simulink model "Nonlinear_Adaptive_Backstepping_controller"  (R2021a)
settings: Solver=VariableStepAuto  StartTime=0.0  StopTime=50  RelTol=1e-3
libraries: simulink x2
settings Model: Creator=dell  LastModifiedBy=dell

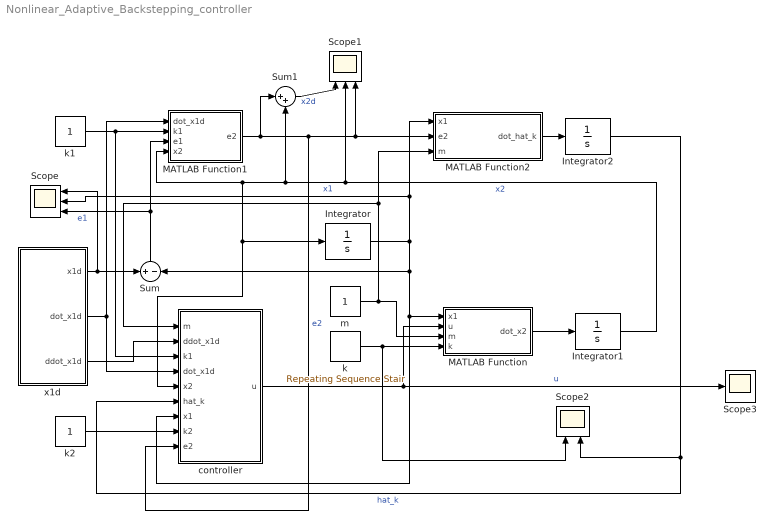
== system Nonlinear_Adaptive_Backstepping_controller ==
  Integrator : Integrator
  Integrator1 : Integrator
  Integrator2 : Integrator
  MATLAB Function : MATLAB Function  TreatAsAtomicUnit=on
  MATLAB Function1 : MATLAB Function  TreatAsAtomicUnit=on
  MATLAB Function2 : MATLAB Function  TreatAsAtomicUnit=on
  Scope : Scope  NumInputPorts=3
  Scope1 : Scope  NumInputPorts=3
  Scope2 : Scope  NumInputPorts=2
  Scope3 : Scope
  Sum : Sum  Inputs=+-
  Sum1 : Sum  Inputs=|++
  controller : MATLAB Function  TreatAsAtomicUnit=on
  k : simulink/Sources/Repeating Sequence Stair  OutValues=[3 1 4 1 5 9 2 6].'  tsamp=25  OutMin=[]  OutMax=[]  OutDataTypeStr=double  OutputDataTypeScalingMode=double  OutDataType=fixdt(0,8)  ConRadixGroup=Best Precision: Vector-wise  OutScaling=2^-12
  k1 : Constant
  k2 : Constant
  m : Constant
  x1d : Subsystem
  wires:
  Integrator/1 -> controller/7(x1), MATLAB Function/1(x1), Sum/2, Scope/2, MATLAB Function2/1(x1)  "x1"
  Integrator1/1 -> Scope1/2, Sum1/2, MATLAB Function1/4(x2), controller/5(x2), Integrator/1  "x2"
  m/1 -> MATLAB Function2/3(m), controller/1(m), MATLAB Function/3(m)
  k/1 -> Scope2/1, MATLAB Function/4(k)
  controller/1(u) -> Scope3/1, MATLAB Function/2(u)  "u"
  MATLAB Function/1(dot_x2) -> Integrator1/1
  x1d/1(x1d) -> Scope/1, Sum/1
  Sum/1 -> Scope/3, MATLAB Function1/3(e1)  "e1"
  x1d/2(dot_x1d) -> controller/4(dot_x1d), MATLAB Function1/1(dot_x1d)
  k1/1 -> MATLAB Function1/2(k1), controller/3(k1)
  MATLAB Function2/1(dot_hat_k) -> Integrator2/1
  Integrator2/1 -> Scope2/2, controller/6(hat_k)  "hat_k"
  MATLAB Function1/1(e2) -> Sum1/1, controller/9(e2), Scope1/3, MATLAB Function2/2(e2)  "e2"
  x1d/3(ddot_x1d) -> controller/2(ddot_x1d)
  k2/1 -> controller/8(k2)
  Sum1/1 -> Scope1/1  "x2d"

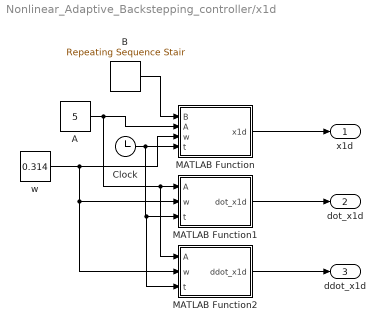
== system Nonlinear_Adaptive_Backstepping_controller/x1d ==
  A : Constant  Value=5
  B : simulink/Sources/Repeating Sequence Stair  OutValues=[0].'  tsamp=10  OutMin=[]  OutMax=[]  OutDataTypeStr=double  OutputDataTypeScalingMode=double  OutDataType=fixdt(0,8)  ConRadixGroup=Best Precision: Vector-wise  OutScaling=2^-12
  Clock : Clock
  MATLAB Function : MATLAB Function  TreatAsAtomicUnit=on
  MATLAB Function1 : MATLAB Function  TreatAsAtomicUnit=on
  MATLAB Function2 : MATLAB Function  TreatAsAtomicUnit=on
  w : Constant  Value=0.314
  x1d : Outport
  dot_x1d : Outport  Port=2
  ddot_x1d : Outport  Port=3
  wires:
  MATLAB Function/1(x1d) -> x1d/1
  Clock/1 -> MATLAB Function2/3(t), MATLAB Function1/3(t), MATLAB Function/4(t)
  B/1 -> MATLAB Function/1(B)
  A/1 -> MATLAB Function2/1(A), MATLAB Function1/1(A), MATLAB Function/2(A)
  w/1 -> MATLAB Function2/2(w), MATLAB Function1/2(w), MATLAB Function/3(w)
  MATLAB Function1/1(dot_x1d) -> dot_x1d/1
  MATLAB Function2/1(ddot_x1d) -> ddot_x1d/1

== matlab function Nonlinear_Adaptive_Backstepping_controller/controller ==
  data: m input; u output; ddot_x1d input; k1 input; dot_x1d input; x2 input; hat_k input; x1 input; k2 input; e2 input
function u = fcn(m,ddot_x1d, k1,dot_x1d,x2,hat_k,x1,k2,e2)

u = m*ddot_x1d+m*k1*(dot_x1d-x2)+hat_k*x1^3+m*k2*e2;

== matlab function Nonlinear_Adaptive_Backstepping_controller/MATLAB Function ==
  data: x1 input; dot_x2 output; u input; m input; k input
function dot_x2 = fcn(x1,u,m,k)

dot_x2 = -k/m*x1^3+1/m*u;

== matlab function Nonlinear_Adaptive_Backstepping_controller/MATLAB Function1 ==
  data: dot_x1d input; e2 output; k1 input; e1 input; x2 input
function e2 = fcn(dot_x1d,k1,e1,x2)

e2 = dot_x1d+k1*e1-x2;

== matlab function Nonlinear_Adaptive_Backstepping_controller/MATLAB Function2 ==
  data: x1 input; dot_hat_k output; e2 input; m input
function dot_hat_k = fcn(x1,e2,m)

dot_hat_k = e2/m*x1^3;

== matlab function Nonlinear_Adaptive_Backstepping_controller/x1d/MATLAB Function ==
  data: B input; x1d output; A input; w input; t input
function x1d = fcn(B,A,w,t)

x1d = B+A*sin(w*t);

== matlab function Nonlinear_Adaptive_Backstepping_controller/x1d/MATLAB Function1 ==
  data: dot_x1d output; A input; w input; t input
function dot_x1d = fcn(A,w,t)

dot_x1d = A*w*cos(w*t);

== matlab function Nonlinear_Adaptive_Backstepping_controller/x1d/MATLAB Function2 ==
  data: ddot_x1d output; A input; w input; t input
function ddot_x1d = fcn(A,w,t)

ddot_x1d = -1*A*w*w*sin(w*t);
